simulink model "Projeto_Final_versao_1_M21"  (R2021a)
settings: Solver=VariableStepAuto  StartTime=0  StopTime=144  FixedStep=0.1  RelTol=1e-3
model workspace (MAT data in the model file):
  N_P0 = 3
  variavelteste = 0
libraries: spsACVoltageSourceLib x1, spsCurrentMeasurementLib x1, spsSeriesRLCBranchLib x1, autolibsharedmappedengines x1, spspowerguiLib x1
(part 4 of 4)

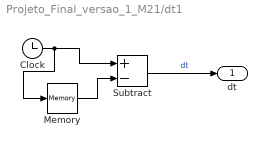
== system Projeto_Final_versao_1_M21/dt1 ==
  Clock : Clock
  Memory : Memory
  Subtract : Sum  Inputs=+-
  dt : Outport
  wires:
  Memory/1 -> Subtract/2
  Clock/1 -> Memory/1, Subtract/1
  Subtract/1 -> dt/1  "dt"

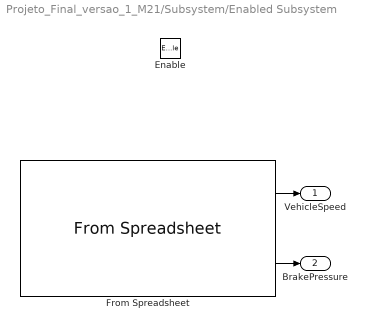
== system Projeto_Final_versao_1_M21/Subsystem/Enabled Subsystem ==
  Enable : EnablePort
  From Spreadsheet : FromSpreadsheet  FileName=C:\Users\Desktop\Downloads\tempo.xlsx  SheetName=tempo  Range=A1:C1441  SampleTime=-1
  VehicleSpeed : Outport  InitialOutput=0  VectorParamsAs1DForOutWhenUnconnected=off
  BrakePressure : Outport  Port=2  InitialOutput=0  VectorParamsAs1DForOutWhenUnconnected=off
  wires:
  From Spreadsheet/1 -> VehicleSpeed/1
  From Spreadsheet/2 -> BrakePressure/1

== stateflow chart Projeto_Final_versao_1_M21/Sistema Ar Condicionado/Chart1 ==
  state AC_Normal
    entry:
    AC_OK = 1;
  state AC_Block
    entry:
    AC_OK = 0;
  (default) -> AC_Normal
  AC_Block -> AC_Normal : [abs(CabinTemperature - TargetTemperature) <= DeltaArCondVAR || (TargetTemperature - CabinTemperature) <= DeltaArCondVAR]
  AC_Normal -> AC_Block : [abs(CabinTemperature - TargetTemperature) > DeltaArCondVAR || (TargetTemperature - CabinTemperature) > DeltaArCondVAR]
  data: CabinTemperature input; TargetTemperature input double; AC_OK output double; DeltaArCondVAR input

== matlab function Projeto_Final_versao_1_M21/Subsystem/MATLAB Function ==
  data: Marcha input; Ativar output; EngineSwitch input
function Ativar = AtivarSubSistema(Marcha, EngineSwitch)
%A marcha igual a 3 significa que o carro está no "D" - Modo Drive

if ((Marcha==3) && (EngineSwitch==1))  
    Ativar = 1;
else 
    Ativar = 0;
end

== stateflow chart Projeto_Final_versao_1_M21/Start Stop/  ==
  state EngineON1
    entry:
    EngineState = 1;  % Motor ligado
    tempo_espera = 0;  % Reseta o contador ao entrar no estado
    during:
    tempo_espera = 0;  % Sempre zera enquanto está no ON normal
  state EngineOFF1
    EngineState = 0;  % Motor desligado
  state WaitToStopAgain
    EngineState = 1;  % Motor ligado
  state WaitForAutoStop
    entry:
    tempo_espera = 0;  % reseta o timer ao entrar
    during:
    tempo_espera = tempo_espera + dt;  % incrementa dt real da simulaçao
  state AutoStop1
    EngineState = 0;  % Motor desligado temporariamente
  EngineON1 -> EngineOFF1 [order 1] : [(EngineSwitch == 0) && (GearPos == 1)]
  EngineOFF1 -> EngineON1 : [EngineSwitch == 1]
  WaitToStopAgain -> EngineON1 [order 1] : [hasChanged(VehicleSpeed)]
  EngineON1 -> WaitForAutoStop [order 2] : [((GearPos == 3) || (GearPos == 2)) && (BrakePressure > BrakePressureVAR) && (VehicleSpeed==VehicleSpeedVAR) && ...
      |  (EngineTemperature > EngineTemperatureVAR) && (AC_OK == 1) && (BattVoltage >= SOC_VAR) && (DoorStatus == 1) && ...
      |  (EPBStatus == 0) &&  (SeatBeltStatus == 1) && (HoodStatus == 1) && (CatalystTemperature > CatalystTemperatureVAR) && ...
      |  (SteeringAngle < SteeringAngleVAR) && (-SteeringAngleVAR < SteeringAngle) && (SteepSlope < SteepSlopeVAR) && (StartStopStatus ==1) ]
  (default) -> EngineOFF1
  WaitToStopAgain -> EngineOFF1 [order 2] : [(EngineSwitch == 0) && (GearPos == 1)]
  AutoStop1 -> WaitToStopAgain : [(BrakePressure < 0.2) || (AC_OK == 0) || (DoorStatus == 0) || (SeatBeltStatus == 0) || (BattVoltage < 12) || (EPBStatus == 1) || (GearPos == 1) || (GearPos == 4) || hasChanged(SteeringAngle)]
  WaitForAutoStop -> AutoStop1 : [tempo_espera >= 1]
  data: BrakePressureVAR input; VehicleSpeedVAR input; EngineTemperatureVAR input; SOC_VAR input; CatalystTemperatureVAR input; SteeringAngleVAR input; SteepSlopeVAR input; VehicleSpeed input; BrakePressure input; THRPEDAL input; SeatBeltStatus input; HoodStatus input; DoorStatus input; GearPos input; EPBStatus input; EngineSwitch input double; tempo_espera local double =0; dt input =0.01; BattVoltage input; EngineTemperature input; AC_OK input; tempoespera local double =0; SteeringAngle input; CatalystTemperature input; SteepSlope input; StartStopStatus input; EngineState output

== matlab function Projeto_Final_versao_1_M21/Subsystem/Inverte Sinal do torque aceleraçãoXdesaceleração ==
  data: EngTrq input; EngTrqSaida output; derivada input
function EngTrqSaida = SinalDoTorque(EngTrq,derivada)

%derivada positiva sinal positivo, derivada negativa sinal de saida
%negativo

if (derivada>0)  
    EngTrqSaida = EngTrq;
else 
    EngTrqSaida = -EngTrq;
end

== matlab function Projeto_Final_versao_1_M21/Câmbio/MATLAB Function1 ==
  data: Marcha input; PosicaoMarcha output; Char output
function [PosicaoMarcha,Char] = ConverterMarcha(Marcha)

if Marcha == 'P'
    PosicaoMarcha = 1; 
    Char = uint8(80);
elseif Marcha == 'N'
    PosicaoMarcha = 2; 
    Char = uint8(78);
elseif Marcha == 'D'
    PosicaoMarcha = 3; 
    Char = uint8(68);
elseif Marcha == 'R'
    PosicaoMarcha = 4; 
    Char = uint8(82);
else 
    PosicaoMarcha = 0;
    Char = uint8(69);
end

== matlab function Projeto_Final_versao_1_M21/MATLAB Function ==
  data: SteeringAngle input; Volante output
function Volante = Dashboard(SteeringAngle)
%#codegen

if ((SteeringAngle < SteeringAngleVAR) && (-SteeringAngleVAR < SteeringAngle))
    Volante = 1;
else
    Volante = 0;
end
